simulink model "PiSquare"  (R2020a)
settings: Solver=FixedStepDiscrete  StartTime=0.0  StopTime=100.0  RelTol=1e-3
undefined symbols (not defined in the file): DiscIntNeverNeededParam
libraries: simulink x1
settings Model: Creator=sadamu  LastModifiedBy=sadamu
settings OptimizationCC: OptimizeBlockIOStorage=off  OptimizeDataStoreBuffers=off  BusAssignmentInplaceUpdate=off
settings DebuggingCC: SFUnexpectedBacktrackingDiag=warning  SFNoUnconditionalDefaultTransitionDiag=warning
settings RTWCC: GenerateReport=on  BuildConfiguration=Debug  LaunchReport=on
settings CodeAppCC: GenerateComments=off  MATLABSourceComments=on  EnableCustomComments=on
settings GRTTargetCC: CombineSignalStateStructs=on  SupportVariableSizeSignals=on  MultiInstanceErrorCode=Warning

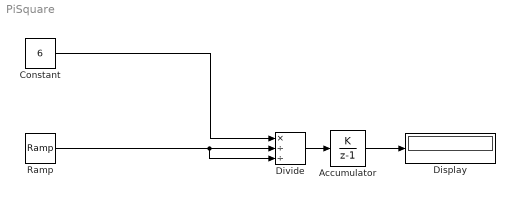
== system PiSquare ==
  Accumulator : DiscreteIntegrator  IntegratorMethod=Accumulation: Forward Euler  ICPrevOutput=DiscIntNeverNeededParam  ICPrevScaledInput=DiscIntNeverNeededParam
  Constant : Constant  Value=6
  Display : Display
  Divide : Product  Inputs=*//
  Ramp : simulink/Sources/Ramp  slope=1  start=0  InitialOutput=1
  wires:
  Divide/1 -> Accumulator/1
  Ramp/1 -> Divide/3, Divide/2
  Constant/1 -> Divide/1
  Accumulator/1 -> Display/1
